simulink library "FUSA_SENSMON"  (R2024b)
settings: Solver=VariableStepAuto  StartTime=0.0  StopTime=10.0  RelTol=1e-3
libraries: simulink x7
settings Model: Creator=jmbsp  LastModifiedBy=jmbsp

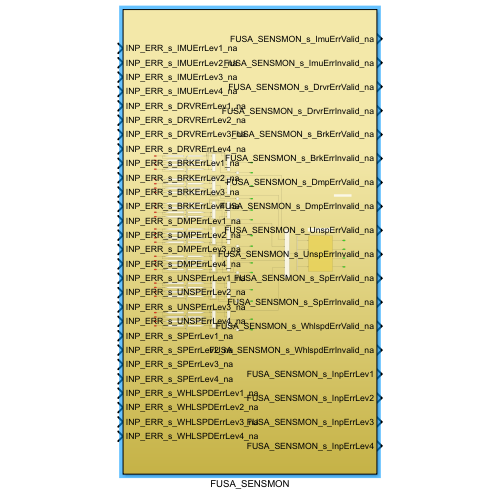
[thumbnail: Simulink's stored preview of the top-level diagram]
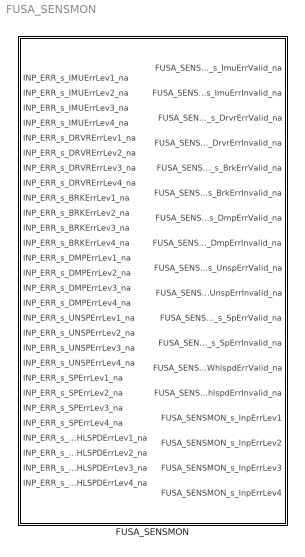
== system FUSA_SENSMON ==
  FUSA_SENSMON : Subsystem

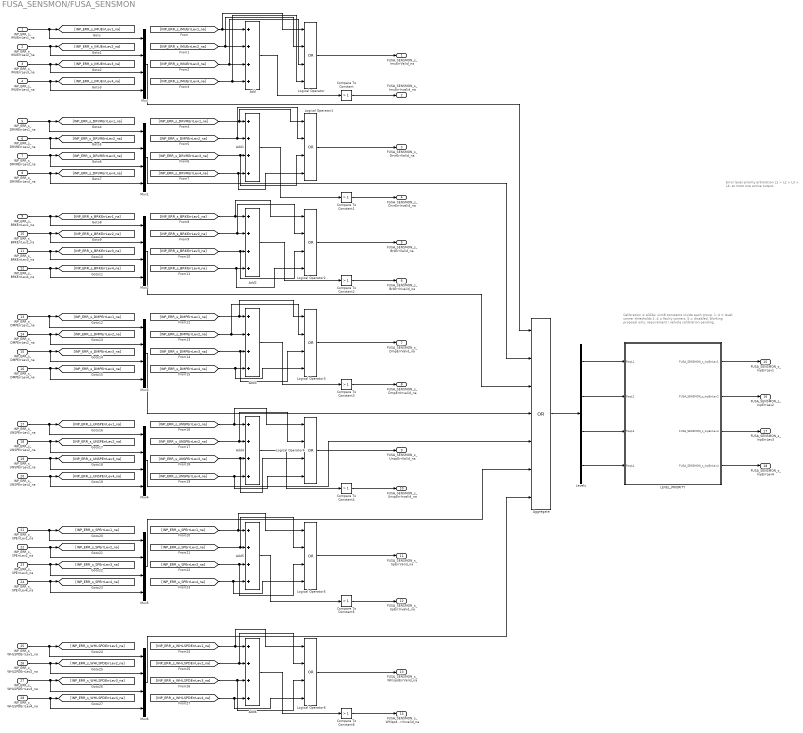
== system FUSA_SENSMON/FUSA_SENSMON ==
  note: Calibration is LOCAL: uint8 constants inside each group.
      | 1..4 = level; corner thresholds 1..4 = faulty corners, 5 = disabled.
      | Working proposal only; requirement / vehicle calibration pending.
  note: Error level priority arbitration
      | L1 > L2 > L3 > L4; at most one active output.
  INP_ERR_s_IMUErrLev1_na : Inport
  INP_ERR_s_IMUErrLev2_na : Inport  Port=2
  INP_ERR_s_IMUErrLev3_na : Inport  Port=3
  INP_ERR_s_IMUErrLev4_na : Inport  Port=4
  INP_ERR_s_DRVRErrLev1_na : Inport  Port=5
  INP_ERR_s_DRVRErrLev2_na : Inport  Port=6
  INP_ERR_s_DRVRErrLev3_na : Inport  Port=7
  INP_ERR_s_DRVRErrLev4_na : Inport  Port=8
  INP_ERR_s_BRKErrLev1_na : Inport  Port=9
  INP_ERR_s_BRKErrLev2_na : Inport  Port=10
  INP_ERR_s_BRKErrLev3_na : Inport  Port=11
  INP_ERR_s_BRKErrLev4_na : Inport  Port=12
  INP_ERR_s_DMPErrLev1_na : Inport  Port=13
  INP_ERR_s_DMPErrLev2_na : Inport  Port=14
  INP_ERR_s_DMPErrLev3_na : Inport  Port=15
  INP_ERR_s_DMPErrLev4_na : Inport  Port=16
  INP_ERR_s_UNSPErrLev1_na : Inport  Port=17
  INP_ERR_s_UNSPErrLev2_na : Inport  Port=18
  INP_ERR_s_UNSPErrLev3_na : Inport  Port=19
  INP_ERR_s_UNSPErrLev4_na : Inport  Port=20
  INP_ERR_s_SPErrLev1_na : Inport  Port=21
  INP_ERR_s_SPErrLev2_na : Inport  Port=22
  INP_ERR_s_SPErrLev3_na : Inport  Port=23
  INP_ERR_s_SPErrLev4_na : Inport  Port=24
  INP_ERR_s_WHLSPDErrLev1_na : Inport  Port=25
  INP_ERR_s_WHLSPDErrLev2_na : Inport  Port=26
  INP_ERR_s_WHLSPDErrLev3_na : Inport  Port=27
  INP_ERR_s_WHLSPDErrLev4_na : Inport  Port=28
  Add{,1..6} (7 alike) : Sum  Inputs=++++
  Aggregate : Logic  Operator=OR  Inputs=7  AllPortsSameDT=off  OutDataTypeStr=boolean
  Compare To Constant{,1..6} (7 alike) : simulink/Logic and Bit Operations/Compare To Constant  relop=>  const=1  OutDataTypeStr=boolean
  LEVEL_PRIORITY : Subsystem
  Levels : Demux
  Logical Operator{,1..6} (7 alike) : Logic  Operator=OR  Inputs=4  AllPortsSameDT=off  OutDataTypeStr=boolean
  Mux{,1..6} (7 alike) : Mux
  FUSA_SENSMON_s_ImuErrValid_na : Outport
  FUSA_SENSMON_s_ImuErrInvalid_na : Outport  Port=2
  FUSA_SENSMON_s_DrvrErrValid_na : Outport  Port=3
  FUSA_SENSMON_s_DrvrErrInvalid_na : Outport  Port=4
  FUSA_SENSMON_s_BrkErrValid_na : Outport  Port=5
  FUSA_SENSMON_s_BrkErrInvalid_na : Outport  Port=6
  FUSA_SENSMON_s_DmpErrValid_na : Outport  Port=7
  FUSA_SENSMON_s_DmpErrInvalid_na : Outport  Port=8
  FUSA_SENSMON_s_UnspErrValid_na : Outport  Port=9
  FUSA_SENSMON_s_UnspErrInvalid_na : Outport  Port=10
  FUSA_SENSMON_s_SpErrValid_na : Outport  Port=11
  FUSA_SENSMON_s_SpErrInvalid_na : Outport  Port=12
  FUSA_SENSMON_s_WhlspdErrValid_na : Outport  Port=13
  FUSA_SENSMON_s_WhlspdErrInvalid_na : Outport  Port=14
  FUSA_SENSMON_s_InpErrLev1 : Outport  Port=15
  FUSA_SENSMON_s_InpErrLev2 : Outport  Port=16
  FUSA_SENSMON_s_InpErrLev3 : Outport  Port=17
  FUSA_SENSMON_s_InpErrLev4 : Outport  Port=18
  wires:
  INP_ERR_s_IMUErrLev1_na/1 -> Mux/1, [INP_ERR_s_IMUErrLev1_na]
  INP_ERR_s_IMUErrLev2_na/1 -> Mux/2, [INP_ERR_s_IMUErrLev2_na]
  INP_ERR_s_IMUErrLev3_na/1 -> Mux/3, [INP_ERR_s_IMUErrLev3_na]
  INP_ERR_s_IMUErrLev4_na/1 -> Mux/4, [INP_ERR_s_IMUErrLev4_na]
  [INP_ERR_s_IMUErrLev4_na] -> Logical Operator/4, Add/4
  [INP_ERR_s_IMUErrLev3_na] -> Logical Operator/3, Add/3
  [INP_ERR_s_IMUErrLev2_na] -> Logical Operator/2, Add/2
  [INP_ERR_s_IMUErrLev1_na] -> Logical Operator/1, Add/1
  [INP_ERR_s_DRVRErrLev1_na] -> Logical Operator1/1, Add1/1
  [INP_ERR_s_DMPErrLev2_na] -> Logical Operator1/2, Add1/2
  [INP_ERR_s_DRVRErrLev3_na] -> Logical Operator1/3, Add1/3
  [INP_ERR_s_DRVRErrLev4_na] -> Logical Operator1/4, Add1/4
  [INP_ERR_s_BRKErrLev1_na] -> Logical Operator2/1, Add2/1
  [INP_ERR_s_BRKErrLev2_na] -> Logical Operator2/2, Add2/2
  [INP_ERR_s_BRKErrLev3_na] -> Logical Operator2/3, Add2/3
  [INP_ERR_s_BRKErrLev4_na] -> Logical Operator2/4, Add2/4
  [INP_ERR_s_DMPErrLev1_na] -> Logical Operator3/1, Add3/1
  [INP_ERR_s_DMPErrLev2_na] -> Logical Operator3/2, Add3/2
  [INP_ERR_s_DMPErrLev3_na] -> Logical Operator3/3, Add3/3
  [INP_ERR_s_DMPErrLev4_na] -> Logical Operator3/4, Add3/4
  [INP_ERR_s_UNSPErrLev1_na] -> Logical Operator4/1, Add4/1
  [INP_ERR_s_UNSPErrLev2_na] -> Logical Operator4/2, Add4/2
  [INP_ERR_s_UNSPErrLev3_na] -> Logical Operator4/3, Add4/3
  [INP_ERR_s_UNSPErrLev4_na] -> Logical Operator4/4, Add4/4
  [INP_ERR_s_SPErrLev1_na] -> Logical Operator5/1, Add5/1
  [INP_ERR_s_SPErrLev2_na] -> Logical Operator5/2, Add5/2
  [INP_ERR_s_SPErrLev3_na] -> Logical Operator5/3, Add5/3
  [INP_ERR_s_SPErrLev4_na] -> Logical Operator5/4, Add5/4
  [INP_ERR_s_WHLSPDErrLev1_na] -> Logical Operator6/1, Add6/1
  [INP_ERR_s_WHLSPDErrLev2_na] -> Logical Operator6/2, Add6/2
  [INP_ERR_s_WHLSPDErrLev3_na] -> Logical Operator6/3, Add6/3
  [INP_ERR_s_WHLSPDErrLev4_na] -> Logical Operator6/4, Add6/4
  Add/1 -> Compare To Constant/1
  Add1/1 -> Compare To Constant1/1
  Add2/1 -> Compare To Constant2/1
  Add6/1 -> Compare To Constant6/1
  Add5/1 -> Compare To Constant5/1
  Add4/1 -> Compare To Constant4/1
  Add3/1 -> Compare To Constant3/1
  Mux3/1 -> Aggregate/4
  Mux1/1 -> Aggregate/2
  Aggregate/1 -> Levels/1
  Mux5/1 -> Aggregate/6
  Mux2/1 -> Aggregate/3
  Mux/1 -> Aggregate/1
  Mux4/1 -> Aggregate/5
  Mux6/1 -> Aggregate/7
  Logical Operator/1 -> FUSA_SENSMON_s_ImuErrValid_na/1
  Compare To Constant/1 -> FUSA_SENSMON_s_ImuErrInvalid_na/1
  Logical Operator1/1 -> FUSA_SENSMON_s_DrvrErrValid_na/1
  Compare To Constant1/1 -> FUSA_SENSMON_s_DrvrErrInvalid_na/1
  Logical Operator2/1 -> FUSA_SENSMON_s_BrkErrValid_na/1
  Compare To Constant2/1 -> FUSA_SENSMON_s_BrkErrInvalid_na/1
  Logical Operator3/1 -> FUSA_SENSMON_s_DmpErrValid_na/1
  Compare To Constant3/1 -> FUSA_SENSMON_s_DmpErrInvalid_na/1
  Logical Operator4/1 -> FUSA_SENSMON_s_UnspErrValid_na/1
  Compare To Constant4/1 -> FUSA_SENSMON_s_UnspErrInvalid_na/1
  Logical Operator5/1 -> FUSA_SENSMON_s_SpErrValid_na/1
  Compare To Constant5/1 -> FUSA_SENSMON_s_SpErrInvalid_na/1
  Logical Operator6/1 -> FUSA_SENSMON_s_WhlspdErrValid_na/1
  Compare To Constant6/1 -> FUSA_SENSMON_s_WhlspdErrInvalid_na/1
  INP_ERR_s_DRVRErrLev1_na/1 -> Mux1/1, [INP_ERR_s_DRVRErrLev1_na]
  INP_ERR_s_DRVRErrLev2_na/1 -> Mux1/2, [INP_ERR_s_DRVRErrLev2_na]
  INP_ERR_s_DRVRErrLev4_na/1 -> Mux1/4, [INP_ERR_s_DRVRErrLev4_na]
  INP_ERR_s_DRVRErrLev3_na/1 -> Mux1/3, [INP_ERR_s_DRVRErrLev3_na]
  INP_ERR_s_BRKErrLev3_na/1 -> Mux2/3, [INP_ERR_s_BRKErrLev3_na]
  INP_ERR_s_BRKErrLev4_na/1 -> Mux2/4, [INP_ERR_s_BRKErrLev4_na]
  INP_ERR_s_BRKErrLev2_na/1 -> Mux2/2, [INP_ERR_s_BRKErrLev2_na]
  INP_ERR_s_BRKErrLev1_na/1 -> Mux2/1, [INP_ERR_s_BRKErrLev1_na]
  INP_ERR_s_DMPErrLev3_na/1 -> Mux3/3, [INP_ERR_s_DMPErrLev3_na]
  INP_ERR_s_DMPErrLev4_na/1 -> Mux3/4, [INP_ERR_s_DMPErrLev4_na]
  INP_ERR_s_DMPErrLev2_na/1 -> Mux3/2, [INP_ERR_s_DMPErrLev2_na]
  INP_ERR_s_DMPErrLev1_na/1 -> Mux3/1, [INP_ERR_s_DMPErrLev1_na]
  INP_ERR_s_UNSPErrLev3_na/1 -> Mux4/3, [INP_ERR_s_UNSPErrLev3_na]
  INP_ERR_s_UNSPErrLev4_na/1 -> Mux4/4, [INP_ERR_s_UNSPErrLev4_na]
  INP_ERR_s_UNSPErrLev2_na/1 -> Mux4/2, [INP_ERR_s_UNSPErrLev2_na]
  INP_ERR_s_UNSPErrLev1_na/1 -> Mux4/1, [INP_ERR_s_UNSPErrLev1_na]
  INP_ERR_s_SPErrLev3_na/1 -> Mux5/3, [INP_ERR_s_SPErrLev3_na]
  INP_ERR_s_SPErrLev4_na/1 -> Mux5/4, [INP_ERR_s_SPErrLev4_na]
  INP_ERR_s_SPErrLev2_na/1 -> Mux5/2, [INP_ERR_s_SPErrLev2_na]
  INP_ERR_s_SPErrLev1_na/1 -> Mux5/1, [INP_ERR_s_SPErrLev1_na]
  INP_ERR_s_WHLSPDErrLev3_na/1 -> Mux6/3, [INP_ERR_s_WHLSPDErrLev3_na]
  INP_ERR_s_WHLSPDErrLev4_na/1 -> Mux6/4, [INP_ERR_s_WHLSPDErrLev4_na]
  INP_ERR_s_WHLSPDErrLev2_na/1 -> Mux6/2, [INP_ERR_s_WHLSPDErrLev2_na]
  INP_ERR_s_WHLSPDErrLev1_na/1 -> Mux6/1, [INP_ERR_s_WHLSPDErrLev1_na]
  Levels/4 -> LEVEL_PRIORITY/4(ReqL4)
  Levels/3 -> LEVEL_PRIORITY/3(ReqL3)
  Levels/2 -> LEVEL_PRIORITY/2(ReqL2)
  Levels/1 -> LEVEL_PRIORITY/1(ReqL1)
  LEVEL_PRIORITY/1(FUSA_SENSMON_s_InpErrLev1) -> FUSA_SENSMON_s_InpErrLev1/1
  LEVEL_PRIORITY/2(FUSA_SENSMON_s_InpErrLev2) -> FUSA_SENSMON_s_InpErrLev2/1
  LEVEL_PRIORITY/3(FUSA_SENSMON_s_InpErrLev3) -> FUSA_SENSMON_s_InpErrLev3/1
  LEVEL_PRIORITY/4(FUSA_SENSMON_s_InpErrLev4) -> FUSA_SENSMON_s_InpErrLev4/1

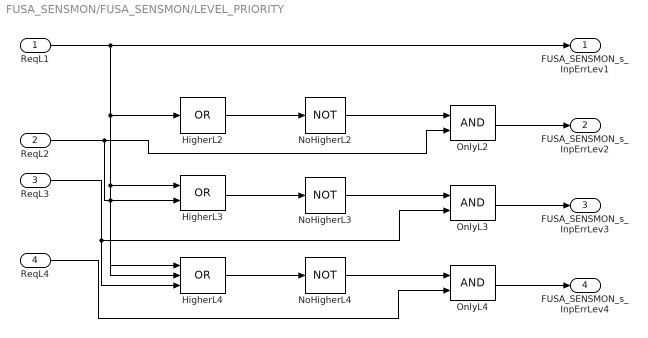
== system FUSA_SENSMON/FUSA_SENSMON/LEVEL_PRIORITY ==
  ReqL1 : Inport  OutDataTypeStr=boolean  PortDimensions=1
  ReqL2 : Inport  Port=2  OutDataTypeStr=boolean  PortDimensions=1
  ReqL3 : Inport  Port=3  OutDataTypeStr=boolean  PortDimensions=1
  ReqL4 : Inport  Port=4  OutDataTypeStr=boolean  PortDimensions=1
  HigherL2 : Logic  Operator=OR  Inputs=1  AllPortsSameDT=off  OutDataTypeStr=boolean
  HigherL3 : Logic  Operator=OR  AllPortsSameDT=off  OutDataTypeStr=boolean
  HigherL4 : Logic  Operator=OR  Inputs=3  AllPortsSameDT=off  OutDataTypeStr=boolean
  NoHigherL2 : Logic  Operator=NOT  Inputs=1  AllPortsSameDT=off  OutDataTypeStr=boolean
  NoHigherL3 : Logic  Operator=NOT  Inputs=1  AllPortsSameDT=off  OutDataTypeStr=boolean
  NoHigherL4 : Logic  Operator=NOT  Inputs=1  AllPortsSameDT=off  OutDataTypeStr=boolean
  OnlyL2 : Logic  AllPortsSameDT=off  OutDataTypeStr=boolean
  OnlyL3 : Logic  AllPortsSameDT=off  OutDataTypeStr=boolean
  OnlyL4 : Logic  AllPortsSameDT=off  OutDataTypeStr=boolean
  FUSA_SENSMON_s_InpErrLev1 : Outport  OutDataTypeStr=boolean
  FUSA_SENSMON_s_InpErrLev2 : Outport  Port=2  OutDataTypeStr=boolean
  FUSA_SENSMON_s_InpErrLev3 : Outport  Port=3  OutDataTypeStr=boolean
  FUSA_SENSMON_s_InpErrLev4 : Outport  Port=4  OutDataTypeStr=boolean
  wires:
  ReqL1/1 -> HigherL3/1, HigherL4/1, HigherL2/1, FUSA_SENSMON_s_InpErrLev1/1
  HigherL2/1 -> NoHigherL2/1
  ReqL2/1 -> OnlyL2/2, HigherL3/2, HigherL4/2
  NoHigherL2/1 -> OnlyL2/1
  OnlyL2/1 -> FUSA_SENSMON_s_InpErrLev2/1
  HigherL3/1 -> NoHigherL3/1
  ReqL3/1 -> OnlyL3/2, HigherL4/3
  NoHigherL3/1 -> OnlyL3/1
  OnlyL3/1 -> FUSA_SENSMON_s_InpErrLev3/1
  HigherL4/1 -> NoHigherL4/1
  ReqL4/1 -> OnlyL4/2
  NoHigherL4/1 -> OnlyL4/1
  OnlyL4/1 -> FUSA_SENSMON_s_InpErrLev4/1
